simulink model "simu"  (R2020b)
settings: Solver=VariableStepAuto  StartTime=0.0  StopTime=20  RelTol=1e-3
values from neighbouring files (symbols this model uses):
  Aa = zeros(n,n)    [TD1.m]
  Te = 0.5    [TD1.m]
undefined symbols (not defined in the file or in its folder): Bb, F4
settings Model: Creator=Etudiants  LastModifiedBy=Etudiants

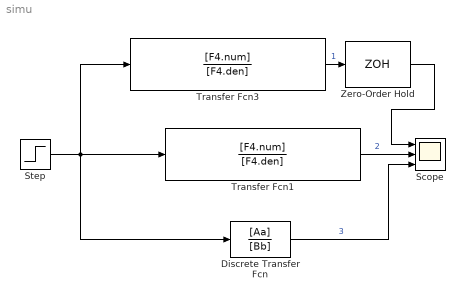
== system simu ==
  Discrete Transfer Fcn : DiscreteTransferFcn  Numerator=[Aa]  Denominator=[Bb]  SampleTime=Te
  Scope : Scope  NumInputPorts=3
  Step : Step  Time=0  After=5  SampleTime=0
  Transfer Fcn1 : TransferFcn  Numerator=[F4.num]  Denominator=[F4.den]
  Transfer Fcn3 : TransferFcn  Numerator=[F4.num]  Denominator=[F4.den]
  Zero-Order Hold : ZeroOrderHold  SampleTime=Te
  wires:
  Step/1 -> Transfer Fcn3/1, Discrete Transfer Fcn/1, Transfer Fcn1/1
  Discrete Transfer Fcn/1 -> Scope/3  "3"
  Transfer Fcn1/1 -> Scope/2  "2"
  Transfer Fcn3/1 -> Zero-Order Hold/1  "1"
  Zero-Order Hold/1 -> Scope/1
